simulink model "assign1cl"  (Simulink 8.6)
settings: Solver=ode45  StartTime=0.0  StopTime=120.0  RelTol=1e-3
values from neighbouring files (symbols this model uses):
  ts = 0.01    [assign1prep.m]
undefined symbols (not defined in the file or in its folder): Cz_den, Cz_num
settings Model: Creator=AartsRGKM  LastModifiedBy=AartsRGKM
settings DataIOCC: SignalLoggingName=sigsOut
settings OptimizationCC: ExpressionDepthLimit=128
settings DebuggingCC: SaveWithParameterizedLinksMsg=none  SignalResolutionControl=TryResolveAllWithWarning  SolverPrmCheckMsg=none  MultiTaskDSMMsg=warning  MultiTaskCondExecSysMsg=none  FcnCallInpInsideContextMsg=EnableAllAsError  StateNameClashWarn=none
settings HardwareCC: TargetUnknown=on
settings GRTTargetCC: GeneratePreprocessorConditionals=Use local settings

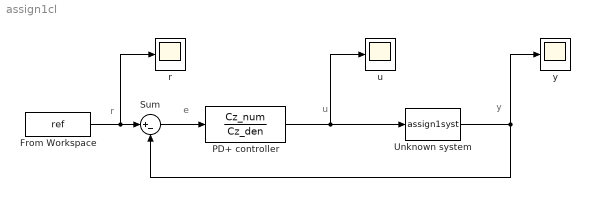
== system assign1cl ==
  note: u
  note: r
  note: e
  note: y
  From Workspace : FromWorkspace  VariableName=ref  SampleTime=0.01  Interpolate=off  OutputAfterFinalValue=Cyclic repetition
  PD+ controller : DiscreteTransferFcn  Numerator=Cz_num  Denominator=Cz_den  SampleTime=ts
  Sum : Sum  Inputs=|+-  SaturateOnIntegerOverflow=on
  Unknown system : M-S-Function  FunctionName=assign1syst
  r : Scope
  u : Scope
  y : Scope
  wires:
  PD+ controller/1 -> Unknown system/1, u/1
  From Workspace/1 -> Sum/1, r/1
  Sum/1 -> PD+ controller/1
  Unknown system/1 -> y/1, Sum/2
